simulink model "c221106_FCEV_SLMP_SQP"  (R2022b)
settings: Solver=FixedStepAuto  StartTime=0.0  StopTime=DrvCycLen  FixedStep=1  RelTol=1e-3
values from neighbouring files (symbols this model uses):
  AccThrshd = 1    [Config_c221112.m]    (also in Config_c221127.m; Config_c221218.m; Config_c230117.m; Config_c230321.m)
  AlphaRampFactor = 8    [Config_c221112.m]    (also in Config_c221127.m; Config_c221218.m; Config_c230117.m; Config_c230321.m)
  Bat_eff_chg_average = 0.969    [FCEV_original_data.mat]
  Bat_eff_dis_average = 0.9632    [FCEV_original_data.mat]
  Bat_end_of_life_percent = 20    [FCEV_original_data.mat]
  Bat_I_chg_max = -120    [FCEV_original_data.mat]
  Bat_I_dis_max = 200    [FCEV_original_data.mat]
  Bat_nom_Ic = 2.5    [FCEV_original_data.mat]
  Bat_nom_SOC = 0.35    [FCEV_original_data.mat]
  Bat_nom_temp_oC = 25    [FCEV_original_data.mat]
  Bat_num_pa = 9    [FCEV_original_data.mat]
  Bat_num_se = 97    [FCEV_original_data.mat]
  Bat_ori_C1_chg_F = [397.526659684 455.660832136 435.08783522 460.845064365 457.605812374 417.289828504 416.373906992 359.741413056 321.561704819 1109.14132554 1165.67733205 1135.97600211 ... (72 elements, 9x8)]    [FCEV_original_data.mat]
  Bat_ori_C1_dis_F = [187.121968588 287.083505726 346.448009002 395.529439835 387.517274826 389.973134196 432.856765051 486.92921923 512.158935268 425.990733989 614.68708868 771.472592368 ... (72 elements, 9x8)]    [FCEV_original_data.mat]
  Bat_ori_C2_chg_F = [8748.48589695 7773.35875681 9404.86567646 8934.73981058 8290.58671366 7592.78422269 7759.44623103 7396.59043829 6151.35152293 16187.7227039 11721.8480541 13157.8579836 ... (72 elements, 9x8)]    [FCEV_original_data.mat]
  Bat_ori_C2_dis_F = [2939.81325553 4590.73311898 5504.93546413 5887.5077374 6534.37836712 7765.46899768 10584.7751706 10372.0508438 9238.72693885 5207.86390693 7911.43744944 8879.62137571 ... (72 elements, 9x8)]    [FCEV_original_data.mat]
  Bat_ori_cap_max_Ah = 20.7    [Config_c221218.m]    (also in Config_c230117.m; Config_c230321.m; FCEV_original_data.mat)
  Bat_ori_dUdt4 = [-0.303773584906 -0.249056603774 -0.115094339623 -0.0396226415094 0.0396226415094 0.0641509433962 0.107547169811 0.111320754717 0.0415094339623 0.0547169811321 0.130188679245]    [FCEV_original_data.mat]
  Bat_ori_R0_chg_O = [0.0771669453735 0.0731809311402 0.0726556782939 0.0729965156794 0.0731758310684 0.0742031005051 0.0721266921026 0.0714211058078 0.0714186176143 0.0374124505155 0.0354566732504 0.0345430657188 ... (72 elements, 9x8)]    [FCEV_original_data.mat]
  Bat_ori_R0_dis_O = [0.0819458671157 0.0812429476608 0.0803749674507 0.0805513601722 0.0838629023857 0.0850797840015 0.0829875518672 0.0826388888889 0.0812514106148 0.0428124986417 0.0424658903711 0.0428572670451 ... (72 elements, 9x8)]    [FCEV_original_data.mat]
  Bat_ori_R1_chg_O = [0.114339870884 0.105392753268 0.104421193553 0.109821896183 0.114868279838 0.123333154908 0.129174812826 0.149917249373 0.174896487845 0.0420560161846 0.0390948352938 0.0370122837364 ... (72 elements, 9x8)]    [FCEV_original_data.mat]
  Bat_ori_R1_dis_O = [0.304806399643 0.213604089624 0.171463520004 0.151183840498 0.140630862434 0.128795299077 0.116857791733 0.112567113582 0.106368362501 0.0943235089866 0.0730697254134 0.0611414736086 ... (72 elements, 9x8)]    [FCEV_original_data.mat]
  Bat_ori_R2_chg_O = [0.134518959939 0.17565045702 0.161100627268 0.189032232545 0.205639040497 0.226170473035 0.223651875822 0.181765694192 0.212966950836 0.073628872144 0.0788540822416 0.0792414571734 ... (72 elements, 9x8)]    [FCEV_original_data.mat]
  Bat_ori_R2_dis_O = [0.354968099904 0.285293035102 0.286338708953 0.298763853987 0.248762838155 0.178586175471 0.129047399775 0.188406991173 0.174494800676 0.131839238891 0.123225430215 0.132069033134 ... (72 elements, 9x8)]    [FCEV_original_data.mat]
  Bat_ori_SOC2 = [0 0.001 0.002 0.003 0.004 0.005 0.006 0.007 0.008 0.009 0.01 0.011 ... (1001 elements, 1x1001)]    [FCEV_original_data.mat]
  Bat_ori_SOC4 = [-0.00598301069999 0.0920117618231 0.190864167279 0.289083557951 0.387343788287 0.485011843502 0.5850485992 0.678163031937 0.774810095565 0.876684636119 0.972739524626]    [FCEV_original_data.mat]
  Bat_ori_Uoc_chg_V = [2.4478 2.54923264342 2.6007 2.6383 2.66953057366 2.69636321708 2.7197 2.74042850391 2.75906114733 2.77619379074 2.792 2.80675907757 ... (1001 elements, 1x1001)]    [FCEV_original_data.mat]
  Bat_ori_Uoc_dis_V = [1.9998 2.03916768329 2.24724374236 2.39700902919 2.48767431602 2.5476 2.5882 2.6202 2.64771773167 2.6719 2.6933 2.71251566192 ... (1001 elements, 1x1001)]    [FCEV_original_data.mat]
  Bat_ori_Uoc_V = [2.2238 2.29420016335 2.42397187118 2.5176545146 2.57860244484 2.62198160854 2.65395 2.68031425195 2.7033894395 2.72404689537 2.74265 2.75963736975 ... (1001 elements, 1x1001)]    [FCEV_original_data.mat]
  Bat_power_max_kW = 50    [FCEV_original_data.mat]
  Bat_power_min_kW = 0    [FCEV_original_data.mat]
  Bat_single_capacity_nom_Ah = 2.3    [FCEV_original_data.mat]
  Bat_SOC_ini = 0.3    [Config_c22100601.m]    (also in Config_c22100701.m; FCEV_original_data.mat = 0.45)
  Bat_SOC_max = 0.9    [FCEV_original_data.mat]
  Bat_SOC_min = 0.3    [FCEV_original_data.mat]
  Bat_temp_amb_oC = 25    [FCEV_original_data.mat]
  Bat_temp_cool_oC = 25    [FCEV_original_data.mat]
  BattSocInit = 0.9    [Config_c221112.m]    (also in Config_c221127.m = 0.3; Config_c221218.m = 0.3; Config_c230117.m = 0.8; Config_c230321.m = 0.8)
  BattSocLowerLimit = 0.25    [Config_c221112.m]    (also in Config_c221127.m = 0.3; Config_c221218.m = 0.3; Config_c230117.m = 0.3; Config_c230321.m = 0.3)
  BattSocUpperLimit = 0.9    [Config_c221112.m]    (also in Config_c221127.m = 0.8; Config_c221218.m = 0.8; Config_c230117.m = 0.8; Config_c230321.m = 0.8)
  BattValuePlaceholder = 0    [Config_c221112.m]
  DCAC_eff = 0.95    [FCEV_original_data.mat]
  DCDC_ori_eff = [0.95 0.96 0.97 0.976 0.98 0.978 0.973 0.962]    [FCEV_original_data.mat]
  DCDC_ori_power_kW = [0 10 20 30 40 50 60 70]    [FCEV_original_data.mat]
  DeAccThrshd = -1    [Config_c221112.m]    (also in Config_c221127.m; Config_c221218.m; Config_c230117.m; Config_c230321.m)
  DrvCycRange = sum(DrvCycVps(:,2))    [Config_c221112.m]    (also in Config_c221127.m; Config_c221218.m; Config_c230117.m; Config_c230321.m)
  FC_ori_eff = [0.1 0.33 0.492 0.533 0.559 0.596 0.591 0.562 0.508]    [FCEV_original_data.mat]
  FC_ori_fuel_rate_gps = [0 0.0505050505051 0.0846883468835 0.117260787992 0.149075730471 0.279642058166 0.423011844332 0.593119810202 0.820209973753]    [FCEV_original_data.mat]
  FC_ori_power_kW = [0 2 5 7.5 10 20 30 40 50]    [FCEV_original_data.mat]
  FC_power_max_kW = 50    [FCEV_original_data.mat]
  FC_power_min_kW = 0    [FCEV_original_data.mat]
  m = Time_sample    [Config_c22100601.m]    (also in Config_c22100701.m)
  MC_eff_brk_average = 0.810578512397    [FCEV_original_data.mat]
  MC_eff_dri_average = 0.810578512397    [FCEV_original_data.mat]
  MC_inertia = 0.06    [FCEV_original_data.mat]
  MC_ori_eff = [0.7 0.78 0.85 0.86 0.81 0.82 0.79 0.78 0.78 0.78 0.78 0.7 ... (231 elements, 11x21)]    [FCEV_original_data.mat]
  MC_ori_power_brk_req_kW = [0 -28.3912930389 -56.7825860779 -85.1738791168 -113.565172156 -141.956465195 -170.347758234 -198.739051273 -227.130344311 -255.52163735 -283.912930389 0 ... (121 elements, 11x11)]    [FCEV_original_data.mat]
  MC_ori_power_dri_req_kW = [0 0 0 0 0 0 0 0 0 0 0 0 ... (121 elements, 11x11)]    [FCEV_original_data.mat]
  MC_ori_spd_rpm = [0 1000 2000 3000 4000 5000 6000 7000 8000 9000 10000]    [FCEV_original_data.mat]
  MC_ori_trq_brk_max_Nm = [-271.1368 -271.1368 -271.1368 -237.5159 -178.1369 -142.4824 -118.7579 -101.8119 -89.0685 -79.172 -71.1734]    [FCEV_original_data.mat]
  MC_ori_trq_brk_Nm = [-271.136848522 -244.02316367 -216.909478817 -189.795793965 -162.682109113 -135.568424261 -108.454739409 -81.3410545565 -54.2273697044 -27.1136848522 0]    [FCEV_original_data.mat]
  MC_ori_trq_dri_max_Nm = [271.1368 271.1368 271.1368 237.5159 178.1369 142.4824 118.7579 101.8119 89.0685 79.172 71.1734]    [FCEV_original_data.mat]
  MC_ori_trq_dri_Nm = [0 27.1136848522 54.2273697044 81.3410545565 108.454739409 135.568424261 162.682109113 189.795793965 216.909478817 244.02316367 271.136848522]    [FCEV_original_data.mat]
  MC_ori_trq_Nm = [-271.136848522 -244.02316367 -216.909478817 -189.795793965 -162.682109113 -135.568424261 -108.454739409 -81.3410545565 -54.2273697044 -27.1136848522 0 27.1136848522 ... (21 elements, 1x21)]    [FCEV_original_data.mat]
  MC_power_max_kW = 75    [FCEV_original_data.mat]
  MC_spd_max_rpm = 10000    [FCEV_original_data.mat]
  MC_spd_min_rpm = 0    [FCEV_original_data.mat]
  MC_spd_scale = 1    [FCEV_original_data.mat]
  MC_trq_scale = 1    [FCEV_original_data.mat]
  MC_U_min_V = 120    [FCEV_original_data.mat]
  PredLen = 5    [Config_c221112.m]    (also in Config_c221127.m; Config_c221218.m; Config_c230117.m; Config_c230321.m)
  Road_u = 0.75    [FCEV_original_data.mat]
  SC_np = 1    [Config_c230321.m]
  SC_ns = 100    [Config_c230321.m]
  SC_rc = 1000    [Config_c230321.m]
  SLMP_LearningRate = 0.05    [Config_c221112.m]    (also in Config_c221127.m; Config_c221218.m; Config_c230117.m; Config_c230321.m)
  usd2rmb = 7.116    [Config_c22100601.m]    (also in Config_c22100701.m; Config_c221106.m = 6; Config_c221112.m = 6; Config_c221127.m = 6)
  Veh_air_density_kgpm2 = 1.2    [FCEV_original_data.mat]
  Veh_brk_front = [1 0.6 0.608 0.61 0.618 0.624 0.636 0.645 0.655]    [FCEV_original_data.mat]
  Veh_brk_z = [0.1 0.2 0.3 0.4 0.5 0.6 0.7 0.8 0.9]    [FCEV_original_data.mat]
  Veh_brk_z_max = 0.7    [FCEV_original_data.mat]
  Veh_brk_z_min = 0.1    [FCEV_original_data.mat]
  Veh_coeff_drag = 0.312    [FCEV_original_data.mat]
  Veh_coeff_roll = 0.00863    [FCEV_original_data.mat]
  Veh_final_drive_inertia = 0.1105    [FCEV_original_data.mat]
  Veh_final_drive_ratio = 3.47    [FCEV_original_data.mat]
  Veh_frontal_area_m2 = 2.06    [FCEV_original_data.mat]
  Veh_gravity_acc_ms2 = 9.81    [FCEV_original_data.mat]
  Veh_mass_cargo_kg = 113    [FCEV_original_data.mat]
  Veh_mass_curb_kg = 1157    [FCEV_original_data.mat]
  Veh_mech_eff = 0.9    [FCEV_original_data.mat]
  Veh_rotary_mass_conversion_factor = 1.05    [FCEV_original_data.mat]
  Veh_size_cg_height_m = 0.53    [FCEV_original_data.mat]
  Veh_wheel_inertia = 3.1039    [FCEV_original_data.mat]
  Veh_wheel_radius_m = 0.313    [FCEV_original_data.mat]
  Veh_wt_frac_front = 0.5    [FCEV_original_data.mat]
  VstdThrshd = 2    [Config_c221112.m]    (also in Config_c221127.m; Config_c221218.m; Config_c230117.m; Config_c230321.m)
undefined symbols (not defined in the file or in its folder): Bat_ori_temp, SC_iv, SC_nm, SC_SocTable
libraries: autolibshared x1
(part 6 of 8)

== system c221106_FCEV_SLMP_SQP/Subsystem4/VehModel_Pred+2/整车动力学模型/坡道阻力 ==
  车辆平均车速1 : Inport
  预测坡度 : Inport  Port=2
  Add : Sum  Inputs=+-
  Add1 : Sum
  Constant : Constant  Value=0
  Constant1 : Constant  Value=Veh_mass_cargo_kg
  Constant2 : Constant  Value=Veh_mass_curb_kg
  Constant3 : Constant  Value=Veh_gravity_acc_ms2
  Fi : Scope
  Memory : Memory  InheritSampleTime=on
  Product : Product  Inputs=3  RndMeth=Zero
  Switch : Switch  SaturateOnIntegerOverflow=off  InputSameDT=off
  Switch1 : Switch  Criteria=u2 > Threshold  SaturateOnIntegerOverflow=off  InputSameDT=off
  Trigonometric Function : Trigonometry  Operator=atan
  Trigonometric Function1 : Trigonometry
  坡道阻力 N : Outport
  wires:
  Trigonometric Function/1 -> Trigonometric Function1/1
  Trigonometric Function1/1 -> Product/1
  Constant3/1 -> Product/3
  Constant/1 -> Switch/3, Switch1/3
  预测坡度/1 -> Trigonometric Function/1
  Switch1/1 -> 坡道阻力 N/1, Fi/1
  Add1/1 -> Product/2
  Constant2/1 -> Add1/1
  Constant1/1 -> Add1/2
  车辆平均车速1/1 -> Add/1, Memory/1, Switch1/2
  Memory/1 -> Add/2
  Product/1 -> Switch/1
  Add/1 -> Switch/2
  Switch/1 -> Switch1/1

== system c221106_FCEV_SLMP_SQP/Subsystem4/VehModel_Pred+2/整车动力学模型/滚动阻力 ==
  车辆平均车速 km/h : Inport
  预测坡度 : Inport  Port=2
  "  1" : Constant  Value=Veh_coeff_roll
  Add : Sum  Inputs=+-
  Add1 : Sum
  Constant : Constant  Value=0
  Constant1 : Constant  Value=Veh_gravity_acc_ms2
  Constant2 : Constant  Value=Veh_mass_curb_kg
  Constant3 : Constant  Value=Veh_mass_cargo_kg
  Fcn1 : Fcn  Expr=atan(u)
  Fcn2 : Fcn  Expr=cos(u)
  Ff : Scope
  Memory : Memory  InheritSampleTime=on
  Product : Product  Inputs=4  RndMeth=Zero
  Switch : Switch  Criteria=u2 > Threshold  SaturateOnIntegerOverflow=off  InputSameDT=off
  Switch1 : Switch  SaturateOnIntegerOverflow=off  InputSameDT=off
  滚动阻力 N : Outport
  wires:
  Fcn2/1 -> Product/3
  Constant/1 -> Switch1/3, Switch/3
  Add1/1 -> Product/1
  Fcn1/1 -> Fcn2/1
  预测坡度/1 -> Fcn1/1
  Constant2/1 -> Add1/1
  Constant3/1 -> Add1/2
  车辆平均车速 km/h/1 -> Switch/2, Memory/1, Add/1
  Switch/1 -> Ff/1, 滚动阻力 N/1
  Constant1/1 -> Product/2
  "  1"/1 -> Product/4
  Product/1 -> Switch1/1
  Memory/1 -> Add/2
  Add/1 -> Switch1/2
  Switch1/1 -> Switch/1

== system c221106_FCEV_SLMP_SQP/Subsystem4/VehModel_Pred+2/整车动力学模型/空气阻力 ==
  veh_spd km/h : Inport
  Add : Sum  Inputs=-+
  Constant : Constant  Value=0
  Constant1 : Constant  Value=Veh_frontal_area_m2
  Constant2 : Constant  Value=Veh_coeff_drag
  Fw : Scope
  Gain : Gain  Gain=1/21.15
  Memory : Memory  InheritSampleTime=on
  Product : Product  Inputs=4  RndMeth=Zero
  Switch : Switch  SaturateOnIntegerOverflow=off  InputSameDT=off
  空气阻力 N : Outport
  wires:
  Constant1/1 -> Product/1
  Constant2/1 -> Product/2
  veh_spd km/h/1 -> Product/3, Memory/1, Add/2, Product/4
  Product/1 -> Gain/1
  Constant/1 -> Switch/3
  Gain/1 -> Switch/1
  Add/1 -> Switch/2
  Memory/1 -> Add/1
  Switch/1 -> Fw/1, 空气阻力 N/1

== system c221106_FCEV_SLMP_SQP/Subsystem4/VehModel_Pred+2/车轮模型/Interia torque ==
  note: This block computes the torque required to overcome the inertia of the
      | wheels and axle.
  车轮线速度 m/s : Inport
  Add : Sum  Inputs=+-
  Constant : Constant  Value=Veh_wheel_inertia
  Constant2 : Constant  Value=0
  Divide : Product  Inputs=**
  Memory : Memory  InheritSampleTime=on
  Switch : Switch  Criteria=u2 > Threshold  SaturateOnIntegerOverflow=off  InputSameDT=off
  axle input speed (rad/s) : Gain  Gain=1/Veh_wheel_radius_m
  inertia torque (Nm) : Outport  InitialOutput=0
  wires:
  Switch/1 -> Divide/1
  Constant/1 -> Divide/2
  Memory/1 -> Add/2
  axle input speed (rad/s)/1 -> Memory/1, Add/1
  车轮线速度 m/s/1 -> axle input speed (rad/s)/1
  Divide/1 -> inertia torque (Nm)/1
  Add/1 -> Switch/1, Switch/2
  Constant2/1 -> Switch/3

== system c221106_FCEV_SLMP_SQP/Subsystem4/VehModel_Pred+2/车轮模型/Interia torque1 ==
  note: This block computes the torque required to overcome the inertia of the
      | wheels and axle.
  车轮线速度 m/s : Inport
  Add : Sum  Inputs=+-
  Add1 : Sum  Inputs=+-
  Clock : Clock
  Constant : Constant  Value=Veh_wheel_inertia
  Constant2 : Constant  Value=0
  Divide : Product  Inputs=**/
  Memory : Memory  InheritSampleTime=on
  Memory1 : Memory  InheritSampleTime=on
  Saturation : Saturate  UpperLimit=1.1  LowerLimit=0.9
  Switch : Switch  SaturateOnIntegerOverflow=off  InputSameDT=off
  axle input speed (rad/s) : Gain  Gain=1/Veh_wheel_radius_m
  inertia torque (Nm) : Outport  InitialOutput=0
  wires:
  Switch/1 -> Divide/1
  Add/1 -> Switch/2, Switch/3
  Constant/1 -> Divide/2
  Memory1/1 -> Add1/2
  Clock/1 -> Memory1/1, Add1/1
  Memory/1 -> Add/2
  axle input speed (rad/s)/1 -> Memory/1, Add/1
  Constant2/1 -> Switch/1
  Add1/1 -> Saturation/1
  Saturation/1 -> Divide/3
  车轮线速度 m/s/1 -> axle input speed (rad/s)/1
  Divide/1 -> inertia torque (Nm)/1

== system c221106_FCEV_SLMP_SQP/Subsystem4/VehModel_Pred+2/驱动电机模型/Brake torque_limited ==
  tor_req nm : Inport
  mc spd rpm : Inport  Port=2
  1-D Lookup Table : Lookup_n-D  NumberOfTableDimensions=1  BreakpointsForDimension1=MC_ori_spd_rpm  Table=MC_ori_trq_brk_max_Nm  RndMeth=Simplest
  MinMax : MinMax  Function=max  Inputs=2
  limted mc torque nm : Outport
  wires:
  tor_req nm/1 -> MinMax/1
  mc spd rpm/1 -> 1-D Lookup Table/1
  1-D Lookup Table/1 -> MinMax/2
  MinMax/1 -> limted mc torque nm/1

== system c221106_FCEV_SLMP_SQP/Subsystem4/VehModel_Pred+2/驱动电机模型/Drive torque_limited ==
  tor_req nm : Inport
  mc spd rpm : Inport  Port=2
  1-D Lookup Table : Lookup_n-D  NumberOfTableDimensions=1  BreakpointsForDimension1=MC_ori_spd_rpm  Table=MC_ori_trq_dri_max_Nm  RndMeth=Simplest
  MinMax : MinMax  Inputs=2
  limted mc torque nm : Outport
  wires:
  tor_req nm/1 -> MinMax/1
  mc spd rpm/1 -> 1-D Lookup Table/1
  1-D Lookup Table/1 -> MinMax/2
  MinMax/1 -> limted mc torque nm/1

== system c221106_FCEV_SLMP_SQP/Subsystem4/VehModel_Pred+2/驱动电机模型/Inertia torque ==
  motor spd rpm : Inport
  Derivative : Derivative
  Gain1 : Gain  Gain=MC_inertia
  rpm->rad/s : Gain  Gain=2*pi/60
  Out1 : Outport
  wires:
  Derivative/1 -> Gain1/1
  Gain1/1 -> Out1/1
  rpm->rad/s/1 -> Derivative/1
  motor spd rpm/1 -> rpm->rad/s/1

== system c221106_FCEV_SLMP_SQP/Subsystem4/VehModel_Pred+2/驱动电机模型/Inertia torque1 ==
  motor spd rpm : Inport
  Derivative : Derivative
  Gain1 : Gain  Gain=MC_inertia
  rpm->rad/s : Gain  Gain=2*pi/60
  Out1 : Outport
  wires:
  Derivative/1 -> Gain1/1
  Gain1/1 -> Out1/1
  rpm->rad/s/1 -> Derivative/1
  motor spd rpm/1 -> rpm->rad/s/1

== system c221106_FCEV_SLMP_SQP/Subsystem4/VehModel_Pred+3/主减及变速器模型/ Effect of inertia (Nm)1 ==
  In1 : Inport
  Constant : Constant  Value=0
  Derivative : Derivative
  Switch : Switch  SaturateOnIntegerOverflow=off  InputSameDT=off
  inertia : Gain  Gain=Veh_final_drive_inertia
  Out1 : Outport
  wires:
  inertia/1 -> Out1/1
  In1/1 -> Derivative/1
  Derivative/1 -> Switch/3, Switch/2
  Constant/1 -> Switch/1
  Switch/1 -> inertia/1

== system c221106_FCEV_SLMP_SQP/Subsystem4/VehModel_Pred+3/主减及变速器模型/Effect of inertia (Nm) ==
  note: The inertia torque is the input torque required to accelerate the
      | final drive's inertia as measured on the input side.
  fd input speed (rad/s) : Inport
  Gain : Gain  Gain=Veh_final_drive_inertia  SaturateOnIntegerOverflow=on  OutDataTypeStr=Inherit: Same as input  ParamDataTypeStr=Inherit: Same as input
  d/dt : Derivative
  drag torque (Nm) : Outport  InitialOutput=0
  wires:
  fd input speed (rad/s)/1 -> d/dt/1
  d/dt/1 -> Gain/1
  Gain/1 -> drag torque (Nm)/1

== system c221106_FCEV_SLMP_SQP/Subsystem4/VehModel_Pred+3/主减及变速器模型/loss (Nm) ==
  note: The loss torque is zero when the gears are not turning,
      | and is applied at the input side of the gear reduction.
  "drive torque (Nm) " : Inport
  Add : Sum  Inputs=+-
  Gain : Gain  Gain=1/Veh_mech_eff
  Gain1 : Gain  Gain=1/Veh_final_drive_ratio
  drag torque (Nm) : Outport  InitialOutput=0
  wires:
  Add/1 -> drag torque (Nm)/1
  "drive torque (Nm) "/1 -> Gain1/1
  Gain1/1 -> Add/2, Gain/1
  Gain/1 -> Add/1

== system c221106_FCEV_SLMP_SQP/Subsystem4/VehModel_Pred+3/主减及变速器模型/loss (Nm)1 ==
  note: The loss torque is zero when the gears are not turning,
      | and is applied at the input side of the gear reduction.
  "drive torque (Nm) " : Inport
  Add : Sum  Inputs=+-
  Gain : Gain  Gain=1/Veh_mech_eff
  Gain1 : Gain  Gain=1/Veh_final_drive_ratio
  drag torque (Nm) : Outport  InitialOutput=0
  wires:
  Add/1 -> drag torque (Nm)/1
  "drive torque (Nm) "/1 -> Gain1/1
  Gain1/1 -> Add/2, Gain/1
  Gain/1 -> Add/1

== system c221106_FCEV_SLMP_SQP/Subsystem4/VehModel_Pred+3/整车动力学模型/compute of front axle brk from motor ==
  平均车速 km/h : Inport
  " security scale" : Constant
  Add2 : Sum  Inputs=+-
  Add3 : Sum
  Constant : Constant  Value=0
  Constant2 : Constant  Value=Veh_mass_curb_kg
  Constant3 : Constant  Value=Veh_mass_cargo_kg
  Memory : Memory  InheritSampleTime=on
  Product : Product  Inputs=3  RndMeth=Zero
  Switch : Switch  Criteria=u2 > Threshold  SaturateOnIntegerOverflow=off  InputSameDT=off
  km/h->m/s : Gain  Gain=1/3.6
  veh_front_axle_motor_brk : Outport
  wires:
  Memory/1 -> Add2/2
  Add2/1 -> Switch/2, km/h->m/s/1
  km/h->m/s/1 -> Switch/3
  Constant/1 -> Switch/1
  Switch/1 -> Product/2
  " security scale"/1 -> Product/3
  Constant2/1 -> Add3/1
  Constant3/1 -> Add3/2
  Add3/1 -> Product/1
  Product/1 -> veh_front_axle_motor_brk/1
  平均车速 km/h/1 -> Add2/1, Memory/1

== system c221106_FCEV_SLMP_SQP/Subsystem4/VehModel_Pred+3/整车动力学模型/加速阻力 ==
  Input1 : Inport
  Input : Inport  Port=2
  Add : Sum  Inputs=+-
  Add2 : Sum
  Constant : Constant  Value=0
  Constant1 : Constant  Value=Veh_rotary_mass_conversion_factor
  Constant2 : Constant  Value=Veh_mass_curb_kg
  Constant3 : Constant  Value=Veh_mass_cargo_kg
  Divide : Product  Inputs=***
  Fj : Scope
  Gain : Gain
  Scope : Scope  NumInputPorts=2
  Switch : Switch  Criteria=u2 > Threshold  SaturateOnIntegerOverflow=off  InputSameDT=off
  km/h->m/s : Gain  Gain=1/3.6
  加速阻力 N : Outport
  wires:
  km/h->m/s/1 -> Switch/2, Divide/2
  Gain/1 -> 加速阻力 N/1, Fj/1
  Add2/1 -> Divide/1
  Constant2/1 -> Add2/1
  Constant3/1 -> Add2/2
  Constant1/1 -> Divide/3
  Divide/1 -> Switch/1
  Constant/1 -> Switch/3
  Switch/1 -> Gain/1
  Add/1 -> km/h->m/s/1
  Input/1 -> Scope/2, Add/2
  Input1/1 -> Scope/1, Add/1

== system c221106_FCEV_SLMP_SQP/Subsystem4/VehModel_Pred+3/整车动力学模型/坡道阻力 ==
  车辆平均车速1 : Inport
  预测坡度 : Inport  Port=2
  Add : Sum  Inputs=+-
  Add1 : Sum
  Constant : Constant  Value=0
  Constant1 : Constant  Value=Veh_mass_cargo_kg
  Constant2 : Constant  Value=Veh_mass_curb_kg
  Constant3 : Constant  Value=Veh_gravity_acc_ms2
  Fi : Scope
  Memory : Memory  InheritSampleTime=on
  Product : Product  Inputs=3  RndMeth=Zero
  Switch : Switch  SaturateOnIntegerOverflow=off  InputSameDT=off
  Switch1 : Switch  Criteria=u2 > Threshold  SaturateOnIntegerOverflow=off  InputSameDT=off
  Trigonometric Function : Trigonometry  Operator=atan
  Trigonometric Function1 : Trigonometry
  坡道阻力 N : Outport
  wires:
  Trigonometric Function/1 -> Trigonometric Function1/1
  Trigonometric Function1/1 -> Product/1
  Constant3/1 -> Product/3
  Constant/1 -> Switch/3, Switch1/3
  预测坡度/1 -> Trigonometric Function/1
  Switch1/1 -> 坡道阻力 N/1, Fi/1
  Add1/1 -> Product/2
  Constant2/1 -> Add1/1
  Constant1/1 -> Add1/2
  车辆平均车速1/1 -> Add/1, Memory/1, Switch1/2
  Memory/1 -> Add/2
  Product/1 -> Switch/1
  Add/1 -> Switch/2
  Switch/1 -> Switch1/1

== system c221106_FCEV_SLMP_SQP/Subsystem4/VehModel_Pred+3/整车动力学模型/滚动阻力 ==
  车辆平均车速 km/h : Inport
  预测坡度 : Inport  Port=2
  "  1" : Constant  Value=Veh_coeff_roll
  Add : Sum  Inputs=+-
  Add1 : Sum
  Constant : Constant  Value=0
  Constant1 : Constant  Value=Veh_gravity_acc_ms2
  Constant2 : Constant  Value=Veh_mass_curb_kg
  Constant3 : Constant  Value=Veh_mass_cargo_kg
  Fcn1 : Fcn  Expr=atan(u)
  Fcn2 : Fcn  Expr=cos(u)
  Ff : Scope
  Memory : Memory  InheritSampleTime=on
  Product : Product  Inputs=4  RndMeth=Zero
  Switch : Switch  Criteria=u2 > Threshold  SaturateOnIntegerOverflow=off  InputSameDT=off
  Switch1 : Switch  SaturateOnIntegerOverflow=off  InputSameDT=off
  滚动阻力 N : Outport
  wires:
  Fcn2/1 -> Product/3
  Constant/1 -> Switch1/3, Switch/3
  Add1/1 -> Product/1
  Fcn1/1 -> Fcn2/1
  预测坡度/1 -> Fcn1/1
  Constant2/1 -> Add1/1
  Constant3/1 -> Add1/2
  车辆平均车速 km/h/1 -> Switch/2, Memory/1, Add/1
  Switch/1 -> Ff/1, 滚动阻力 N/1
  Constant1/1 -> Product/2
  "  1"/1 -> Product/4
  Product/1 -> Switch1/1
  Memory/1 -> Add/2
  Add/1 -> Switch1/2
  Switch1/1 -> Switch/1

== system c221106_FCEV_SLMP_SQP/Subsystem4/VehModel_Pred+3/整车动力学模型/空气阻力 ==
  veh_spd km/h : Inport
  Add : Sum  Inputs=-+
  Constant : Constant  Value=0
  Constant1 : Constant  Value=Veh_frontal_area_m2
  Constant2 : Constant  Value=Veh_coeff_drag
  Fw : Scope
  Gain : Gain  Gain=1/21.15
  Memory : Memory  InheritSampleTime=on
  Product : Product  Inputs=4  RndMeth=Zero
  Switch : Switch  SaturateOnIntegerOverflow=off  InputSameDT=off
  空气阻力 N : Outport
  wires:
  Constant1/1 -> Product/1
  Constant2/1 -> Product/2
  veh_spd km/h/1 -> Product/3, Memory/1, Add/2, Product/4
  Product/1 -> Gain/1
  Constant/1 -> Switch/3
  Gain/1 -> Switch/1
  Add/1 -> Switch/2
  Memory/1 -> Add/1
  Switch/1 -> Fw/1, 空气阻力 N/1

== system c221106_FCEV_SLMP_SQP/Subsystem4/VehModel_Pred+3/车轮模型/Interia torque ==
  note: This block computes the torque required to overcome the inertia of the
      | wheels and axle.
  车轮线速度 m/s : Inport
  Add : Sum  Inputs=+-
  Constant : Constant  Value=Veh_wheel_inertia
  Constant2 : Constant  Value=0
  Divide : Product  Inputs=**
  Memory : Memory  InheritSampleTime=on
  Switch : Switch  Criteria=u2 > Threshold  SaturateOnIntegerOverflow=off  InputSameDT=off
  axle input speed (rad/s) : Gain  Gain=1/Veh_wheel_radius_m
  inertia torque (Nm) : Outport  InitialOutput=0
  wires:
  Switch/1 -> Divide/1
  Constant/1 -> Divide/2
  Memory/1 -> Add/2
  axle input speed (rad/s)/1 -> Memory/1, Add/1
  车轮线速度 m/s/1 -> axle input speed (rad/s)/1
  Divide/1 -> inertia torque (Nm)/1
  Add/1 -> Switch/1, Switch/2
  Constant2/1 -> Switch/3

== system c221106_FCEV_SLMP_SQP/Subsystem4/VehModel_Pred+3/车轮模型/Interia torque1 ==
  note: This block computes the torque required to overcome the inertia of the
      | wheels and axle.
  车轮线速度 m/s : Inport
  Add : Sum  Inputs=+-
  Add1 : Sum  Inputs=+-
  Clock : Clock
  Constant : Constant  Value=Veh_wheel_inertia
  Constant2 : Constant  Value=0
  Divide : Product  Inputs=**/
  Memory : Memory  InheritSampleTime=on
  Memory1 : Memory  InheritSampleTime=on
  Saturation : Saturate  UpperLimit=1.1  LowerLimit=0.9
  Switch : Switch  SaturateOnIntegerOverflow=off  InputSameDT=off
  axle input speed (rad/s) : Gain  Gain=1/Veh_wheel_radius_m
  inertia torque (Nm) : Outport  InitialOutput=0
  wires:
  Switch/1 -> Divide/1
  Add/1 -> Switch/2, Switch/3
  Constant/1 -> Divide/2
  Memory1/1 -> Add1/2
  Clock/1 -> Memory1/1, Add1/1
  Memory/1 -> Add/2
  axle input speed (rad/s)/1 -> Memory/1, Add/1
  Constant2/1 -> Switch/1
  Add1/1 -> Saturation/1
  Saturation/1 -> Divide/3
  车轮线速度 m/s/1 -> axle input speed (rad/s)/1
  Divide/1 -> inertia torque (Nm)/1

== system c221106_FCEV_SLMP_SQP/Subsystem4/VehModel_Pred+3/驱动电机模型/Brake torque_limited ==
  tor_req nm : Inport
  mc spd rpm : Inport  Port=2
  1-D Lookup Table : Lookup_n-D  NumberOfTableDimensions=1  BreakpointsForDimension1=MC_ori_spd_rpm  Table=MC_ori_trq_brk_max_Nm  RndMeth=Simplest
  MinMax : MinMax  Function=max  Inputs=2
  limted mc torque nm : Outport
  wires:
  tor_req nm/1 -> MinMax/1
  mc spd rpm/1 -> 1-D Lookup Table/1
  1-D Lookup Table/1 -> MinMax/2
  MinMax/1 -> limted mc torque nm/1

== system c221106_FCEV_SLMP_SQP/Subsystem4/VehModel_Pred+3/驱动电机模型/Drive torque_limited ==
  tor_req nm : Inport
  mc spd rpm : Inport  Port=2
  1-D Lookup Table : Lookup_n-D  NumberOfTableDimensions=1  BreakpointsForDimension1=MC_ori_spd_rpm  Table=MC_ori_trq_dri_max_Nm  RndMeth=Simplest
  MinMax : MinMax  Inputs=2
  limted mc torque nm : Outport
  wires:
  tor_req nm/1 -> MinMax/1
  mc spd rpm/1 -> 1-D Lookup Table/1
  1-D Lookup Table/1 -> MinMax/2
  MinMax/1 -> limted mc torque nm/1

== system c221106_FCEV_SLMP_SQP/Subsystem4/VehModel_Pred+3/驱动电机模型/Inertia torque ==
  motor spd rpm : Inport
  Derivative : Derivative
  Gain1 : Gain  Gain=MC_inertia
  rpm->rad/s : Gain  Gain=2*pi/60
  Out1 : Outport
  wires:
  Derivative/1 -> Gain1/1
  Gain1/1 -> Out1/1
  rpm->rad/s/1 -> Derivative/1
  motor spd rpm/1 -> rpm->rad/s/1

== system c221106_FCEV_SLMP_SQP/Subsystem4/VehModel_Pred+3/驱动电机模型/Inertia torque1 ==
  motor spd rpm : Inport
  Derivative : Derivative
  Gain1 : Gain  Gain=MC_inertia
  rpm->rad/s : Gain  Gain=2*pi/60
  Out1 : Outport
  wires:
  Derivative/1 -> Gain1/1
  Gain1/1 -> Out1/1
  rpm->rad/s/1 -> Derivative/1
  motor spd rpm/1 -> rpm->rad/s/1

== system c221106_FCEV_SLMP_SQP/Subsystem4/VehModel_Pred+4/主减及变速器模型/ Effect of inertia (Nm)1 ==
  In1 : Inport
  Constant : Constant  Value=0
  Derivative : Derivative
  Switch : Switch  SaturateOnIntegerOverflow=off  InputSameDT=off
  inertia : Gain  Gain=Veh_final_drive_inertia
  Out1 : Outport
  wires:
  inertia/1 -> Out1/1
  In1/1 -> Derivative/1
  Derivative/1 -> Switch/3, Switch/2
  Constant/1 -> Switch/1
  Switch/1 -> inertia/1

== system c221106_FCEV_SLMP_SQP/Subsystem4/VehModel_Pred+4/主减及变速器模型/Effect of inertia (Nm) ==
  note: The inertia torque is the input torque required to accelerate the
      | final drive's inertia as measured on the input side.
  fd input speed (rad/s) : Inport
  Gain : Gain  Gain=Veh_final_drive_inertia  SaturateOnIntegerOverflow=on  OutDataTypeStr=Inherit: Same as input  ParamDataTypeStr=Inherit: Same as input
  d/dt : Derivative
  drag torque (Nm) : Outport  InitialOutput=0
  wires:
  fd input speed (rad/s)/1 -> d/dt/1
  d/dt/1 -> Gain/1
  Gain/1 -> drag torque (Nm)/1

== system c221106_FCEV_SLMP_SQP/Subsystem4/VehModel_Pred+4/主减及变速器模型/loss (Nm) ==
  note: The loss torque is zero when the gears are not turning,
      | and is applied at the input side of the gear reduction.
  "drive torque (Nm) " : Inport
  Add : Sum  Inputs=+-
  Gain : Gain  Gain=1/Veh_mech_eff
  Gain1 : Gain  Gain=1/Veh_final_drive_ratio
  drag torque (Nm) : Outport  InitialOutput=0
  wires:
  Add/1 -> drag torque (Nm)/1
  "drive torque (Nm) "/1 -> Gain1/1
  Gain1/1 -> Add/2, Gain/1
  Gain/1 -> Add/1

== system c221106_FCEV_SLMP_SQP/Subsystem4/VehModel_Pred+4/主减及变速器模型/loss (Nm)1 ==
  note: The loss torque is zero when the gears are not turning,
      | and is applied at the input side of the gear reduction.
  "drive torque (Nm) " : Inport
  Add : Sum  Inputs=+-
  Gain : Gain  Gain=1/Veh_mech_eff
  Gain1 : Gain  Gain=1/Veh_final_drive_ratio
  drag torque (Nm) : Outport  InitialOutput=0
  wires:
  Add/1 -> drag torque (Nm)/1
  "drive torque (Nm) "/1 -> Gain1/1
  Gain1/1 -> Add/2, Gain/1
  Gain/1 -> Add/1

== system c221106_FCEV_SLMP_SQP/Subsystem4/VehModel_Pred+4/整车动力学模型/compute of front axle brk from motor ==
  平均车速 km/h : Inport
  " security scale" : Constant
  Add2 : Sum  Inputs=+-
  Add3 : Sum
  Constant : Constant  Value=0
  Constant2 : Constant  Value=Veh_mass_curb_kg
  Constant3 : Constant  Value=Veh_mass_cargo_kg
  Memory : Memory  InheritSampleTime=on
  Product : Product  Inputs=3  RndMeth=Zero
  Switch : Switch  Criteria=u2 > Threshold  SaturateOnIntegerOverflow=off  InputSameDT=off
  km/h->m/s : Gain  Gain=1/3.6
  veh_front_axle_motor_brk : Outport
  wires:
  Memory/1 -> Add2/2
  Add2/1 -> Switch/2, km/h->m/s/1
  km/h->m/s/1 -> Switch/3
  Constant/1 -> Switch/1
  Switch/1 -> Product/2
  " security scale"/1 -> Product/3
  Constant2/1 -> Add3/1
  Constant3/1 -> Add3/2
  Add3/1 -> Product/1
  Product/1 -> veh_front_axle_motor_brk/1
  平均车速 km/h/1 -> Add2/1, Memory/1

== system c221106_FCEV_SLMP_SQP/Subsystem4/VehModel_Pred+4/整车动力学模型/加速阻力 ==
  车速 km/h : Inport
  车速 km/h1 : Inport  Port=2
  Add : Sum  Inputs=+-
  Add2 : Sum
  Constant : Constant  Value=0
  Constant1 : Constant  Value=Veh_rotary_mass_conversion_factor
  Constant2 : Constant  Value=Veh_mass_curb_kg
  Constant3 : Constant  Value=Veh_mass_cargo_kg
  Divide : Product  Inputs=***
  Fj : Scope
  Gain : Gain
  Switch : Switch  Criteria=u2 > Threshold  SaturateOnIntegerOverflow=off  InputSameDT=off
  km/h->m/s : Gain  Gain=1/3.6
  加速阻力 N : Outport
  wires:
  km/h->m/s/1 -> Switch/2, Divide/2
  Gain/1 -> 加速阻力 N/1, Fj/1
  Add2/1 -> Divide/1
  Constant2/1 -> Add2/1
  Constant3/1 -> Add2/2
  Constant1/1 -> Divide/3
  Divide/1 -> Switch/1
  Constant/1 -> Switch/3
  Switch/1 -> Gain/1
  Add/1 -> km/h->m/s/1
  车速 km/h1/1 -> Add/2
  车速 km/h/1 -> Add/1

== system c221106_FCEV_SLMP_SQP/Subsystem4/VehModel_Pred+4/整车动力学模型/坡道阻力 ==
  车辆平均车速1 : Inport
  预测坡度 : Inport  Port=2
  Add : Sum  Inputs=+-
  Add1 : Sum
  Constant : Constant  Value=0
  Constant1 : Constant  Value=Veh_mass_cargo_kg
  Constant2 : Constant  Value=Veh_mass_curb_kg
  Constant3 : Constant  Value=Veh_gravity_acc_ms2
  Fi : Scope
  Memory : Memory  InheritSampleTime=on
  Product : Product  Inputs=3  RndMeth=Zero
  Switch : Switch  SaturateOnIntegerOverflow=off  InputSameDT=off
  Switch1 : Switch  Criteria=u2 > Threshold  SaturateOnIntegerOverflow=off  InputSameDT=off
  Trigonometric Function : Trigonometry  Operator=atan
  Trigonometric Function1 : Trigonometry
  坡道阻力 N : Outport
  wires:
  Trigonometric Function/1 -> Trigonometric Function1/1
  Trigonometric Function1/1 -> Product/1
  Constant3/1 -> Product/3
  Constant/1 -> Switch/3, Switch1/3
  预测坡度/1 -> Trigonometric Function/1
  Switch1/1 -> 坡道阻力 N/1, Fi/1
  Add1/1 -> Product/2
  Constant2/1 -> Add1/1
  Constant1/1 -> Add1/2
  车辆平均车速1/1 -> Add/1, Memory/1, Switch1/2
  Memory/1 -> Add/2
  Product/1 -> Switch/1
  Add/1 -> Switch/2
  Switch/1 -> Switch1/1

== system c221106_FCEV_SLMP_SQP/Subsystem4/VehModel_Pred+4/整车动力学模型/滚动阻力 ==
  车辆平均车速 km/h : Inport
  预测坡度 : Inport  Port=2
  "  1" : Constant  Value=Veh_coeff_roll
  Add : Sum  Inputs=+-
  Add1 : Sum
  Constant : Constant  Value=0
  Constant1 : Constant  Value=Veh_gravity_acc_ms2
  Constant2 : Constant  Value=Veh_mass_curb_kg
  Constant3 : Constant  Value=Veh_mass_cargo_kg
  Fcn1 : Fcn  Expr=atan(u)
  Fcn2 : Fcn  Expr=cos(u)
  Ff : Scope
  Memory : Memory  InheritSampleTime=on
  Product : Product  Inputs=4  RndMeth=Zero
  Switch : Switch  Criteria=u2 > Threshold  SaturateOnIntegerOverflow=off  InputSameDT=off
  Switch1 : Switch  SaturateOnIntegerOverflow=off  InputSameDT=off
  滚动阻力 N : Outport
  wires:
  Fcn2/1 -> Product/3
  Constant/1 -> Switch1/3, Switch/3
  Add1/1 -> Product/1
  Fcn1/1 -> Fcn2/1
  预测坡度/1 -> Fcn1/1
  Constant2/1 -> Add1/1
  Constant3/1 -> Add1/2
  车辆平均车速 km/h/1 -> Switch/2, Memory/1, Add/1
  Switch/1 -> Ff/1, 滚动阻力 N/1
  Constant1/1 -> Product/2
  "  1"/1 -> Product/4
  Product/1 -> Switch1/1
  Memory/1 -> Add/2
  Add/1 -> Switch1/2
  Switch1/1 -> Switch/1

== system c221106_FCEV_SLMP_SQP/Subsystem4/VehModel_Pred+4/整车动力学模型/空气阻力 ==
  veh_spd km/h : Inport
  Add : Sum  Inputs=-+
  Constant : Constant  Value=0
  Constant1 : Constant  Value=Veh_frontal_area_m2
  Constant2 : Constant  Value=Veh_coeff_drag
  Fw : Scope
  Gain : Gain  Gain=1/21.15
  Memory : Memory  InheritSampleTime=on
  Product : Product  Inputs=4  RndMeth=Zero
  Switch : Switch  SaturateOnIntegerOverflow=off  InputSameDT=off
  空气阻力 N : Outport
  wires:
  Constant1/1 -> Product/1
  Constant2/1 -> Product/2
  veh_spd km/h/1 -> Product/3, Memory/1, Add/2, Product/4
  Product/1 -> Gain/1
  Constant/1 -> Switch/3
  Gain/1 -> Switch/1
  Add/1 -> Switch/2
  Memory/1 -> Add/1
  Switch/1 -> Fw/1, 空气阻力 N/1

== system c221106_FCEV_SLMP_SQP/Subsystem4/VehModel_Pred+4/车轮模型/Interia torque ==
  note: This block computes the torque required to overcome the inertia of the
      | wheels and axle.
  车轮线速度 m/s : Inport
  Add : Sum  Inputs=+-
  Constant : Constant  Value=Veh_wheel_inertia
  Constant2 : Constant  Value=0
  Divide : Product  Inputs=**
  Memory : Memory  InheritSampleTime=on
  Switch : Switch  Criteria=u2 > Threshold  SaturateOnIntegerOverflow=off  InputSameDT=off
  axle input speed (rad/s) : Gain  Gain=1/Veh_wheel_radius_m
  inertia torque (Nm) : Outport  InitialOutput=0
  wires:
  Switch/1 -> Divide/1
  Constant/1 -> Divide/2
  Memory/1 -> Add/2
  axle input speed (rad/s)/1 -> Memory/1, Add/1
  车轮线速度 m/s/1 -> axle input speed (rad/s)/1
  Divide/1 -> inertia torque (Nm)/1
  Add/1 -> Switch/1, Switch/2
  Constant2/1 -> Switch/3

== system c221106_FCEV_SLMP_SQP/Subsystem4/VehModel_Pred+4/车轮模型/Interia torque1 ==
  note: This block computes the torque required to overcome the inertia of the
      | wheels and axle.
  车轮线速度 m/s : Inport
  Add : Sum  Inputs=+-
  Add1 : Sum  Inputs=+-
  Clock : Clock
  Constant : Constant  Value=Veh_wheel_inertia
  Constant2 : Constant  Value=0
  Divide : Product  Inputs=**/
  Memory : Memory  InheritSampleTime=on
  Memory1 : Memory  InheritSampleTime=on
  Saturation : Saturate  UpperLimit=1.1  LowerLimit=0.9
  Switch : Switch  SaturateOnIntegerOverflow=off  InputSameDT=off
  axle input speed (rad/s) : Gain  Gain=1/Veh_wheel_radius_m
  inertia torque (Nm) : Outport  InitialOutput=0
  wires:
  Switch/1 -> Divide/1
  Add/1 -> Switch/2, Switch/3
  Constant/1 -> Divide/2
  Memory1/1 -> Add1/2
  Clock/1 -> Memory1/1, Add1/1
  Memory/1 -> Add/2
  axle input speed (rad/s)/1 -> Memory/1, Add/1
  Constant2/1 -> Switch/1
  Add1/1 -> Saturation/1
  Saturation/1 -> Divide/3
  车轮线速度 m/s/1 -> axle input speed (rad/s)/1
  Divide/1 -> inertia torque (Nm)/1

== system c221106_FCEV_SLMP_SQP/Subsystem4/VehModel_Pred+4/驱动电机模型/Brake torque_limited ==
  tor_req nm : Inport
  mc spd rpm : Inport  Port=2
  1-D Lookup Table : Lookup_n-D  NumberOfTableDimensions=1  BreakpointsForDimension1=MC_ori_spd_rpm  Table=MC_ori_trq_brk_max_Nm  RndMeth=Simplest
  MinMax : MinMax  Function=max  Inputs=2
  limted mc torque nm : Outport
  wires:
  tor_req nm/1 -> MinMax/1
  mc spd rpm/1 -> 1-D Lookup Table/1
  1-D Lookup Table/1 -> MinMax/2
  MinMax/1 -> limted mc torque nm/1

== system c221106_FCEV_SLMP_SQP/Subsystem4/VehModel_Pred+4/驱动电机模型/Drive torque_limited ==
  tor_req nm : Inport
  mc spd rpm : Inport  Port=2
  1-D Lookup Table : Lookup_n-D  NumberOfTableDimensions=1  BreakpointsForDimension1=MC_ori_spd_rpm  Table=MC_ori_trq_dri_max_Nm  RndMeth=Simplest
  MinMax : MinMax  Inputs=2
  limted mc torque nm : Outport
  wires:
  tor_req nm/1 -> MinMax/1
  mc spd rpm/1 -> 1-D Lookup Table/1
  1-D Lookup Table/1 -> MinMax/2
  MinMax/1 -> limted mc torque nm/1

== system c221106_FCEV_SLMP_SQP/Subsystem4/VehModel_Pred+4/驱动电机模型/Inertia torque ==
  motor spd rpm : Inport
  Derivative : Derivative
  Gain1 : Gain  Gain=MC_inertia
  rpm->rad/s : Gain  Gain=2*pi/60
  Out1 : Outport
  wires:
  Derivative/1 -> Gain1/1
  Gain1/1 -> Out1/1
  rpm->rad/s/1 -> Derivative/1
  motor spd rpm/1 -> rpm->rad/s/1

== system c221106_FCEV_SLMP_SQP/Subsystem4/VehModel_Pred+4/驱动电机模型/Inertia torque1 ==
  motor spd rpm : Inport
  Derivative : Derivative
  Gain1 : Gain  Gain=MC_inertia
  rpm->rad/s : Gain  Gain=2*pi/60
  Out1 : Outport
  wires:
  Derivative/1 -> Gain1/1
  Gain1/1 -> Out1/1
  rpm->rad/s/1 -> Derivative/1
  motor spd rpm/1 -> rpm->rad/s/1

== system c221106_FCEV_SLMP_SQP/Subsystem4/VehModel_Pred+5/主减及变速器模型/ Effect of inertia (Nm)1 ==
  In1 : Inport
  Constant : Constant  Value=0
  Derivative : Derivative
  Switch : Switch  SaturateOnIntegerOverflow=off  InputSameDT=off
  inertia : Gain  Gain=Veh_final_drive_inertia
  Out1 : Outport
  wires:
  inertia/1 -> Out1/1
  In1/1 -> Derivative/1
  Derivative/1 -> Switch/3, Switch/2
  Constant/1 -> Switch/1
  Switch/1 -> inertia/1

== system c221106_FCEV_SLMP_SQP/Subsystem4/VehModel_Pred+5/主减及变速器模型/Effect of inertia (Nm) ==
  note: The inertia torque is the input torque required to accelerate the
      | final drive's inertia as measured on the input side.
  fd input speed (rad/s) : Inport
  Gain : Gain  Gain=Veh_final_drive_inertia  SaturateOnIntegerOverflow=on  OutDataTypeStr=Inherit: Same as input  ParamDataTypeStr=Inherit: Same as input
  d/dt : Derivative
  drag torque (Nm) : Outport  InitialOutput=0
  wires:
  fd input speed (rad/s)/1 -> d/dt/1
  d/dt/1 -> Gain/1
  Gain/1 -> drag torque (Nm)/1

== system c221106_FCEV_SLMP_SQP/Subsystem4/VehModel_Pred+5/主减及变速器模型/loss (Nm) ==
  note: The loss torque is zero when the gears are not turning,
      | and is applied at the input side of the gear reduction.
  "drive torque (Nm) " : Inport
  Add : Sum  Inputs=+-
  Gain : Gain  Gain=1/Veh_mech_eff
  Gain1 : Gain  Gain=1/Veh_final_drive_ratio
  drag torque (Nm) : Outport  InitialOutput=0
  wires:
  Add/1 -> drag torque (Nm)/1
  "drive torque (Nm) "/1 -> Gain1/1
  Gain1/1 -> Add/2, Gain/1
  Gain/1 -> Add/1

== system c221106_FCEV_SLMP_SQP/Subsystem4/VehModel_Pred+5/主减及变速器模型/loss (Nm)1 ==
  note: The loss torque is zero when the gears are not turning,
      | and is applied at the input side of the gear reduction.
  "drive torque (Nm) " : Inport
  Add : Sum  Inputs=+-
  Gain : Gain  Gain=1/Veh_mech_eff
  Gain1 : Gain  Gain=1/Veh_final_drive_ratio
  drag torque (Nm) : Outport  InitialOutput=0
  wires:
  Add/1 -> drag torque (Nm)/1
  "drive torque (Nm) "/1 -> Gain1/1
  Gain1/1 -> Add/2, Gain/1
  Gain/1 -> Add/1

== system c221106_FCEV_SLMP_SQP/Subsystem4/VehModel_Pred+5/整车动力学模型/compute of front axle brk from motor ==
  平均车速 km/h : Inport
  " security scale" : Constant
  Add2 : Sum  Inputs=+-
  Add3 : Sum
  Constant : Constant  Value=0
  Constant2 : Constant  Value=Veh_mass_curb_kg
  Constant3 : Constant  Value=Veh_mass_cargo_kg
  Memory : Memory  InheritSampleTime=on
  Product : Product  Inputs=3  RndMeth=Zero
  Switch : Switch  Criteria=u2 > Threshold  SaturateOnIntegerOverflow=off  InputSameDT=off
  km/h->m/s : Gain  Gain=1/3.6
  veh_front_axle_motor_brk : Outport
  wires:
  Memory/1 -> Add2/2
  Add2/1 -> Switch/2, km/h->m/s/1
  km/h->m/s/1 -> Switch/3
  Constant/1 -> Switch/1
  Switch/1 -> Product/2
  " security scale"/1 -> Product/3
  Constant2/1 -> Add3/1
  Constant3/1 -> Add3/2
  Add3/1 -> Product/1
  Product/1 -> veh_front_axle_motor_brk/1
  平均车速 km/h/1 -> Add2/1, Memory/1

== system c221106_FCEV_SLMP_SQP/Subsystem4/VehModel_Pred+5/整车动力学模型/加速阻力 ==
  车速 km/h : Inport
  车速 km/h1 : Inport  Port=2
  Add : Sum  Inputs=+-
  Add2 : Sum
  Constant : Constant  Value=0
  Constant1 : Constant  Value=Veh_rotary_mass_conversion_factor
  Constant2 : Constant  Value=Veh_mass_curb_kg
  Constant3 : Constant  Value=Veh_mass_cargo_kg
  Divide : Product  Inputs=***
  Fj : Scope
  Gain : Gain
  Switch : Switch  Criteria=u2 > Threshold  SaturateOnIntegerOverflow=off  InputSameDT=off
  km/h->m/s : Gain  Gain=1/3.6
  加速阻力 N : Outport
  wires:
  km/h->m/s/1 -> Switch/2, Divide/2
  Gain/1 -> 加速阻力 N/1, Fj/1
  Add2/1 -> Divide/1
  Constant2/1 -> Add2/1
  Constant3/1 -> Add2/2
  Constant1/1 -> Divide/3
  Divide/1 -> Switch/1
  Constant/1 -> Switch/3
  Switch/1 -> Gain/1
  Add/1 -> km/h->m/s/1
  车速 km/h/1 -> Add/1
  车速 km/h1/1 -> Add/2

== system c221106_FCEV_SLMP_SQP/Subsystem4/VehModel_Pred+5/整车动力学模型/坡道阻力 ==
  车辆平均车速1 : Inport
  预测坡度 : Inport  Port=2
  Add : Sum  Inputs=+-
  Add1 : Sum
  Constant : Constant  Value=0
  Constant1 : Constant  Value=Veh_mass_cargo_kg
  Constant2 : Constant  Value=Veh_mass_curb_kg
  Constant3 : Constant  Value=Veh_gravity_acc_ms2
  Fi : Scope
  Memory : Memory  InheritSampleTime=on
  Product : Product  Inputs=3  RndMeth=Zero
  Switch : Switch  SaturateOnIntegerOverflow=off  InputSameDT=off
  Switch1 : Switch  Criteria=u2 > Threshold  SaturateOnIntegerOverflow=off  InputSameDT=off
  Trigonometric Function : Trigonometry  Operator=atan
  Trigonometric Function1 : Trigonometry
  坡道阻力 N : Outport
  wires:
  Trigonometric Function/1 -> Trigonometric Function1/1
  Trigonometric Function1/1 -> Product/1
  Constant3/1 -> Product/3
  Constant/1 -> Switch/3, Switch1/3
  预测坡度/1 -> Trigonometric Function/1
  Switch1/1 -> 坡道阻力 N/1, Fi/1
  Add1/1 -> Product/2
  Constant2/1 -> Add1/1
  Constant1/1 -> Add1/2
  车辆平均车速1/1 -> Add/1, Memory/1, Switch1/2
  Memory/1 -> Add/2
  Product/1 -> Switch/1
  Add/1 -> Switch/2
  Switch/1 -> Switch1/1

== system c221106_FCEV_SLMP_SQP/Subsystem4/VehModel_Pred+5/整车动力学模型/滚动阻力 ==
  车辆平均车速 km/h : Inport
  预测坡度 : Inport  Port=2
  "  1" : Constant  Value=Veh_coeff_roll
  Add : Sum  Inputs=+-
  Add1 : Sum
  Constant : Constant  Value=0
  Constant1 : Constant  Value=Veh_gravity_acc_ms2
  Constant2 : Constant  Value=Veh_mass_curb_kg
  Constant3 : Constant  Value=Veh_mass_cargo_kg
  Fcn1 : Fcn  Expr=atan(u)
  Fcn2 : Fcn  Expr=cos(u)
  Ff : Scope
  Memory : Memory  InheritSampleTime=on
  Product : Product  Inputs=4  RndMeth=Zero
  Switch : Switch  Criteria=u2 > Threshold  SaturateOnIntegerOverflow=off  InputSameDT=off
  Switch1 : Switch  SaturateOnIntegerOverflow=off  InputSameDT=off
  滚动阻力 N : Outport
  wires:
  Fcn2/1 -> Product/3
  Constant/1 -> Switch1/3, Switch/3
  Add1/1 -> Product/1
  Fcn1/1 -> Fcn2/1
  预测坡度/1 -> Fcn1/1
  Constant2/1 -> Add1/1
  Constant3/1 -> Add1/2
  车辆平均车速 km/h/1 -> Switch/2, Memory/1, Add/1
  Switch/1 -> Ff/1, 滚动阻力 N/1
  Constant1/1 -> Product/2
  "  1"/1 -> Product/4
  Product/1 -> Switch1/1
  Memory/1 -> Add/2
  Add/1 -> Switch1/2
  Switch1/1 -> Switch/1

== system c221106_FCEV_SLMP_SQP/Subsystem4/VehModel_Pred+5/整车动力学模型/空气阻力 ==
  veh_spd km/h : Inport
  Add : Sum  Inputs=-+
  Constant : Constant  Value=0
  Constant1 : Constant  Value=Veh_frontal_area_m2
  Constant2 : Constant  Value=Veh_coeff_drag
  Fw : Scope
  Gain : Gain  Gain=1/21.15
  Memory : Memory  InheritSampleTime=on
  Product : Product  Inputs=4  RndMeth=Zero
  Switch : Switch  SaturateOnIntegerOverflow=off  InputSameDT=off
  空气阻力 N : Outport
  wires:
  Constant1/1 -> Product/1
  Constant2/1 -> Product/2
  veh_spd km/h/1 -> Product/3, Memory/1, Add/2, Product/4
  Product/1 -> Gain/1
  Constant/1 -> Switch/3
  Gain/1 -> Switch/1
  Add/1 -> Switch/2
  Memory/1 -> Add/1
  Switch/1 -> Fw/1, 空气阻力 N/1

== system c221106_FCEV_SLMP_SQP/Subsystem4/VehModel_Pred+5/车轮模型/Interia torque ==
  note: This block computes the torque required to overcome the inertia of the
      | wheels and axle.
  车轮线速度 m/s : Inport
  Add : Sum  Inputs=+-
  Constant : Constant  Value=Veh_wheel_inertia
  Constant2 : Constant  Value=0
  Divide : Product  Inputs=**
  Memory : Memory  InheritSampleTime=on
  Switch : Switch  Criteria=u2 > Threshold  SaturateOnIntegerOverflow=off  InputSameDT=off
  axle input speed (rad/s) : Gain  Gain=1/Veh_wheel_radius_m
  inertia torque (Nm) : Outport  InitialOutput=0
  wires:
  Switch/1 -> Divide/1
  Constant/1 -> Divide/2
  Memory/1 -> Add/2
  axle input speed (rad/s)/1 -> Memory/1, Add/1
  车轮线速度 m/s/1 -> axle input speed (rad/s)/1
  Divide/1 -> inertia torque (Nm)/1
  Add/1 -> Switch/1, Switch/2
  Constant2/1 -> Switch/3

== system c221106_FCEV_SLMP_SQP/Subsystem4/VehModel_Pred+5/车轮模型/Interia torque1 ==
  note: This block computes the torque required to overcome the inertia of the
      | wheels and axle.
  车轮线速度 m/s : Inport
  Add : Sum  Inputs=+-
  Add1 : Sum  Inputs=+-
  Clock : Clock
  Constant : Constant  Value=Veh_wheel_inertia
  Constant2 : Constant  Value=0
  Divide : Product  Inputs=**/
  Memory : Memory  InheritSampleTime=on
  Memory1 : Memory  InheritSampleTime=on
  Saturation : Saturate  UpperLimit=1.1  LowerLimit=0.9
  Switch : Switch  SaturateOnIntegerOverflow=off  InputSameDT=off
  axle input speed (rad/s) : Gain  Gain=1/Veh_wheel_radius_m
  inertia torque (Nm) : Outport  InitialOutput=0
  wires:
  Switch/1 -> Divide/1
  Add/1 -> Switch/2, Switch/3
  Constant/1 -> Divide/2
  Memory1/1 -> Add1/2
  Clock/1 -> Memory1/1, Add1/1
  Memory/1 -> Add/2
  axle input speed (rad/s)/1 -> Memory/1, Add/1
  Constant2/1 -> Switch/1
  Add1/1 -> Saturation/1
  Saturation/1 -> Divide/3
  车轮线速度 m/s/1 -> axle input speed (rad/s)/1
  Divide/1 -> inertia torque (Nm)/1

== system c221106_FCEV_SLMP_SQP/Subsystem4/VehModel_Pred+5/驱动电机模型/Brake torque_limited ==
  tor_req nm : Inport
  mc spd rpm : Inport  Port=2
  1-D Lookup Table : Lookup_n-D  NumberOfTableDimensions=1  BreakpointsForDimension1=MC_ori_spd_rpm  Table=MC_ori_trq_brk_max_Nm  RndMeth=Simplest
  MinMax : MinMax  Function=max  Inputs=2
  limted mc torque nm : Outport
  wires:
  tor_req nm/1 -> MinMax/1
  mc spd rpm/1 -> 1-D Lookup Table/1
  1-D Lookup Table/1 -> MinMax/2
  MinMax/1 -> limted mc torque nm/1

== system c221106_FCEV_SLMP_SQP/Subsystem4/VehModel_Pred+5/驱动电机模型/Drive torque_limited ==
  tor_req nm : Inport
  mc spd rpm : Inport  Port=2
  1-D Lookup Table : Lookup_n-D  NumberOfTableDimensions=1  BreakpointsForDimension1=MC_ori_spd_rpm  Table=MC_ori_trq_dri_max_Nm  RndMeth=Simplest
  MinMax : MinMax  Inputs=2
  limted mc torque nm : Outport
  wires:
  tor_req nm/1 -> MinMax/1
  mc spd rpm/1 -> 1-D Lookup Table/1
  1-D Lookup Table/1 -> MinMax/2
  MinMax/1 -> limted mc torque nm/1

== system c221106_FCEV_SLMP_SQP/Subsystem4/VehModel_Pred+5/驱动电机模型/Inertia torque ==
  motor spd rpm : Inport
  Derivative : Derivative
  Gain1 : Gain  Gain=MC_inertia
  rpm->rad/s : Gain  Gain=2*pi/60
  Out1 : Outport
  wires:
  Derivative/1 -> Gain1/1
  Gain1/1 -> Out1/1
  rpm->rad/s/1 -> Derivative/1
  motor spd rpm/1 -> rpm->rad/s/1

== system c221106_FCEV_SLMP_SQP/Subsystem4/VehModel_Pred+5/驱动电机模型/Inertia torque1 ==
  motor spd rpm : Inport
  Derivative : Derivative
  Gain1 : Gain  Gain=MC_inertia
  rpm->rad/s : Gain  Gain=2*pi/60
  Out1 : Outport
  wires:
  Derivative/1 -> Gain1/1
  Gain1/1 -> Out1/1
  rpm->rad/s/1 -> Derivative/1
  motor spd rpm/1 -> rpm->rad/s/1

== system c221106_FCEV_SLMP_SQP/Subsystem4/VehModel_Pred+6/主减及变速器模型/ Effect of inertia (Nm)1 ==
  In1 : Inport
  Constant : Constant  Value=0
  Derivative : Derivative
  Switch : Switch  SaturateOnIntegerOverflow=off  InputSameDT=off
  inertia : Gain  Gain=Veh_final_drive_inertia
  Out1 : Outport
  wires:
  Switch/1 -> inertia/1
  Constant/1 -> Switch/1
  Derivative/1 -> Switch/2, Switch/3
  In1/1 -> Derivative/1
  inertia/1 -> Out1/1

== system c221106_FCEV_SLMP_SQP/Subsystem4/VehModel_Pred+6/主减及变速器模型/Effect of inertia (Nm) ==
  note: The inertia torque is the input torque required to accelerate the
      | final drive's inertia as measured on the input side.
  fd input speed (rad/s) : Inport
  Gain : Gain  Gain=Veh_final_drive_inertia  SaturateOnIntegerOverflow=on  OutDataTypeStr=Inherit: Same as input  ParamDataTypeStr=Inherit: Same as input
  d/dt : Derivative
  drag torque (Nm) : Outport  InitialOutput=0
  wires:
  Gain/1 -> drag torque (Nm)/1
  d/dt/1 -> Gain/1
  fd input speed (rad/s)/1 -> d/dt/1

== system c221106_FCEV_SLMP_SQP/Subsystem4/VehModel_Pred+6/主减及变速器模型/loss (Nm) ==
  note: The loss torque is zero when the gears are not turning,
      | and is applied at the input side of the gear reduction.
  "drive torque (Nm) " : Inport
  Add : Sum  Inputs=+-
  Gain : Gain  Gain=1/Veh_mech_eff
  Gain1 : Gain  Gain=1/Veh_final_drive_ratio
  drag torque (Nm) : Outport  InitialOutput=0
  wires:
  Gain/1 -> Add/1
  Gain1/1 -> Gain/1, Add/2
  "drive torque (Nm) "/1 -> Gain1/1
  Add/1 -> drag torque (Nm)/1
